simulink model "sync_baseline"  (R2025b)
settings: Solver=VariableStepAuto  StartTime=0.0  StopTime=10.0  RelTol=1e-3
values from neighbouring files (symbols this model uses):
  Dm = 1e-3    (= 0.001)    [foc_controlsystem_param.m]    (also in motor_param.m)
  Ki_id = wc_c*Rs    (= 380)    [foc_controlsystem_param.m]    (also in motor_param.m)
  Ki_iq = wc_c*Rs    (= 380)    [foc_controlsystem_param.m]    (also in motor_param.m)
  Ki_s = 0.041    [foc_controlsystem_param.m]    (also in motor_param.m)
  Kp_id = wc_c*Ld    (= 10)    [foc_controlsystem_param.m]    (also in motor_param.m)
  Kp_iq = wc_c*Lq    (= 20)    [foc_controlsystem_param.m]    (also in motor_param.m)
  Kp_s = 0.0014    [foc_controlsystem_param.m]    (also in motor_param.m)
  Ld = 0.01    [foc_controlsystem_param.m]    (also in motor_param.m)
  Lq = 0.02    [foc_controlsystem_param.m]    (also in motor_param.m)
  p = 2    [foc_controlsystem_param.m]    (also in motor_param.m)
  Phi = 0.1    [foc_controlsystem_param.m]    (also in motor_param.m)
libraries: fl_lib x60, nesl_utility x60, slpidlib x18, ee_lib x18, eeTransforms x12
(part 5 of 5)

== system sync_baseline/Subsystem5/Controller/FOC/VelocityController ==
  wmref : Inport
  wm : Inport  Port=2
  Gain : Gain  Gain=1/(3/2*p*Phi)
  PIDController : slpidlib/PID Controller  Controller=PI  Form=Parallel  TimeDomain=Continuous-time  UseExternalTs=off  SampleTime=-1  IntegratorMethod=Forward Euler  FilterMethod=Forward Euler  ControllerParametersSource=internal  P=Kp_s  I=Ki_s  UseKiTs=off  D=0  UseExternalDerivativeSource=off  N=100  UseFilter=on  TunerSelectOption=Transfer Function Based (PID Tuner App)  InitialConditionSource=internal  InitialConditionForIntegrator=0  InitialConditionForFilter=0  DifferentiatorICPrevScaledInput=0  ExternalReset=none  TrackingMode=off  Kt=1  LimitOutput=off  SatLimitsSource=internal  UpperSaturationLimit=inf  LowerSaturationLimit=-inf  LinearizeAsGain=on  AntiWindupMode=none  Kb=1  LimitIntegrator=off  UpperIntegratorSaturationLimit=inf  LowerIntegratorSaturationLimit=-inf  POutMin=[]  POutMax=[]  IOutMin=[]  IOutMax=[]  DOutMin=[]  DOutMax=[]  NOutMin=[]  NOutMax=[]  SumOutMin=[]  SumOutMax=[]  SaturationOutMin=[]  SaturationOutMax=[]  PParamMin=[]  PParamMax=[]  IParamMin=[]  IParamMax=[]  DParamMin=[]  DParamMax=[]  NParamMin=[]  NParamMax=[]  KbParamMin=[]  KbParamMax=[]  KtParamMin=[]  KtParamMax=[]  KbOutMin=[]  KbOutMax=[]  KtOutMin=[]  KtOutMax=[]  IntegratorOutMin=[]  IntegratorOutMax=[]  FilterOutMin=[]  FilterOutMax=[]  SumI1OutMin=[]  SumI1OutMax=[]  SumI2OutMin=[]  SumI2OutMax=[]  SumI3OutMin=[]  SumI3OutMax=[]  SumI4OutMin=[]  SumI4OutMax=[]  SumDOutMin=[]  SumDOutMax=[]  DifferentiatorOutMin=[]  DifferentiatorOutMax=[]  FilterDiffOutCoefMin=[]  FilterDiffOutCoefMax=[]  ReciprocalOutMin=[]  ReciprocalOutMax=[]  SumDenOutMin=[]  SumDenOutMax=[]  SumNumOutMin=[]  SumNumOutMax=[]  DivideOutMin=[]  DivideOutMax=[]  UdiffTsProdOutMin=[]  UdiffTsProdOutMax=[]  NTsProdOutMin=[]  NTsProdOutMax=[]  UintegralTsProdOutMin=[]  UintegralTsProdOutMax=[]  UngainTsProdOutMin=[]  UngainTsProdOutMax=[]  ClampingZeroOutDataTypeStr=Inherit: Inherit via back propagation  ClampingZeroOutMin=[]  ClampingZeroOutMax=[]  FilterDenConstantOutDataTypeStr=Inherit: Inherit via back propagation  FilterDenConstantOutMin=[]  FilterDenConstantOutMax=[]  PCopyOutDataTypeStr=Inherit: Inherit via back propagation  PCopyOutMin=[]  PCopyOutMax=[]  NCopyOutDataTypeStr=Inherit: Inherit via back propagation  NCopyOutMin=[]  NCopyOutMax=[]  IntegratorContinuousStateAttributes=''  IntegratorStateMustResolveToSignalObject=off  IntegratorRTWStateStorageClass=Auto  FilterContinuousStateAttributes=''  FilterStateMustResolveToSignalObject=off  FilterRTWStateStorageClass=Auto  ParallelPVariant=InternalParameters  IdealPVariant=Disabled  IVariant=InternalParameters  DVariant=Disabled  IntegratorVariant=Continuous  SatVariant=Disabled  AWVariant=Passthrough  PCopyVariant=Disabled  TRVariant=Disabled  FdbkBlocksVariant=Forward  IdealPFdbkVariant=Disabled  SatFdbkVariant=Disabled  DerivativeFilterVariant=Disabled  NVariant=Disabled  NCopyVariant=Disabled_SignalSpec  FilterICVariant=Disabled  IntegratorICVariant=InternalICs  ExternalResetVariant=Disabled  TRSumVariant=Passthrough  SumFdbkVariant=Disabled  SumVariant=Sum_PI  TsampFilterVariant=InternalTs  TsampNgainVariant=Passthrough  TsampIntegralVariant=Disabled_SignalSpec  ExternalSaturationOutDataTypeStr=Inherit: Same as second input  DerivativeSourceVariant=Disabled  PreIntVariant=InternalPreInt
  Sum : Sum  Inputs=|+-
  Iqref : Outport  VectorParamsAs1DForOutWhenUnconnected=off
  wires:
  PIDController/1 -> Gain/1
  Gain/1 -> Iqref/1
  wmref/1 -> Sum/1
  Sum/1 -> PIDController/1
  wm/1 -> Sum/2

== system sync_baseline/Subsystem5/Controller/FOC/abc2dq ==
  Iabc : Inport
  thetae : Inport  Port=2
  Demux1 : Demux  Outputs=3
  Park Transform : eeTransforms/Park Transform  AxisAlignment=D-axis  PowerInvariant=off
  Terminator : Terminator
  Id : Outport  VectorParamsAs1DForOutWhenUnconnected=off
  Iq : Outport  Port=2  VectorParamsAs1DForOutWhenUnconnected=off
  wires:
  Iabc/1 -> Park Transform/1
  thetae/1 -> Park Transform/2
  Demux1/3 -> Terminator/1
  Park Transform/1 -> Demux1/1
  Demux1/1 -> Id/1
  Demux1/2 -> Iq/1

== system sync_baseline/Subsystem5/Controller/FOC/dq2abc ==
  Vd : Inport
  Vq : Inport  Port=2
  thetae : Inport  Port=3
  Constant : Constant  Value=0
  Inverse Park Transform : eeTransforms/Inverse Park Transform  AxisAlignment=D-axis  PowerInvariant=off
  Mux : Mux  Inputs=3
  Vabc : Outport  VectorParamsAs1DForOutWhenUnconnected=off
  wires:
  thetae/1 -> Inverse Park Transform/2
  Constant/1 -> Mux/3
  Mux/1 -> Inverse Park Transform/1
  Vd/1 -> Mux/1
  Inverse Park Transform/1 -> Vabc/1
  Vq/1 -> Mux/2

== system sync_baseline/Subsystem5/Controller/FOC/thm2the ==
  thm : Inport
  Constant : Constant  Value=2*pi
  Mod : Math  Operator=mod  SignedPower=on
  PolePairs : Gain  Gain=p
  the : Outport  VectorParamsAs1DForOutWhenUnconnected=off
  wires:
  Constant/1 -> Mod/2
  PolePairs/1 -> Mod/1
  Mod/1 -> the/1
  thm/1 -> PolePairs/1

== system sync_baseline/Subsystem5/Controller/FOC/wm2we ==
  wm : Inport
  PolePairs : Gain  Gain=p
  we : Outport  VectorParamsAs1DForOutWhenUnconnected=off
  wires:
  wm/1 -> PolePairs/1
  PolePairs/1 -> we/1

== system sync_baseline/Subsystem/Controller/FOC/CurrentController/Decoupling ==
  note: VdFF = -Lq*Iq*we
  note: VqFF = Ld*Id*we + Phi*we
  Id : Inport
  Iq : Inport  Port=2
  we : Inport  Port=3
  Constant : Constant  Value=Lq
  Constant1 : Constant  Value=Ld
  Constant2 : Constant  Value=Phi
  Gain1 : Gain  Gain=-1
  Product{,1..3} (4 alike) : Product
  Sum : Sum  Inputs=|++
  VdFF : Outport  VectorParamsAs1DForOutWhenUnconnected=off
  VqFF : Outport  Port=2  VectorParamsAs1DForOutWhenUnconnected=off
  wires:
  we/1 -> Product3/2, Product2/2
  Product1/1 -> Sum/1
  Constant2/1 -> Sum/2
  Sum/1 -> Product2/1
  Constant1/1 -> Product1/2
  Id/1 -> Product1/1
  Iq/1 -> Product/1
  Constant/1 -> Product/2
  Product3/1 -> Gain1/1
  Product/1 -> Product3/1
  Gain1/1 -> VdFF/1
  Product2/1 -> VqFF/1

== system sync_baseline/Subsystem1/Controller/FOC/CurrentController/Decoupling ==
  note: VdFF = -Lq*Iq*we
  note: VqFF = Ld*Id*we + Phi*we
  Id : Inport
  Iq : Inport  Port=2
  we : Inport  Port=3
  Constant : Constant  Value=Lq
  Constant1 : Constant  Value=Ld
  Constant2 : Constant  Value=Phi
  Gain1 : Gain  Gain=-1
  Product{,1..3} (4 alike) : Product
  Sum : Sum  Inputs=|++
  VdFF : Outport  VectorParamsAs1DForOutWhenUnconnected=off
  VqFF : Outport  Port=2  VectorParamsAs1DForOutWhenUnconnected=off
  wires:
  we/1 -> Product3/2, Product2/2
  Product1/1 -> Sum/1
  Constant2/1 -> Sum/2
  Sum/1 -> Product2/1
  Constant1/1 -> Product1/2
  Id/1 -> Product1/1
  Iq/1 -> Product/1
  Constant/1 -> Product/2
  Product3/1 -> Gain1/1
  Product/1 -> Product3/1
  Gain1/1 -> VdFF/1
  Product2/1 -> VqFF/1

== system sync_baseline/Subsystem2/Controller/FOC/CurrentController/Decoupling ==
  note: VdFF = -Lq*Iq*we
  note: VqFF = Ld*Id*we + Phi*we
  Id : Inport
  Iq : Inport  Port=2
  we : Inport  Port=3
  Constant : Constant  Value=Lq
  Constant1 : Constant  Value=Ld
  Constant2 : Constant  Value=Phi
  Gain1 : Gain  Gain=-1
  Product{,1..3} (4 alike) : Product
  Sum : Sum  Inputs=|++
  VdFF : Outport  VectorParamsAs1DForOutWhenUnconnected=off
  VqFF : Outport  Port=2  VectorParamsAs1DForOutWhenUnconnected=off
  wires:
  we/1 -> Product3/2, Product2/2
  Product1/1 -> Sum/1
  Constant2/1 -> Sum/2
  Sum/1 -> Product2/1
  Constant1/1 -> Product1/2
  Id/1 -> Product1/1
  Iq/1 -> Product/1
  Constant/1 -> Product/2
  Product3/1 -> Gain1/1
  Product/1 -> Product3/1
  Gain1/1 -> VdFF/1
  Product2/1 -> VqFF/1

== system sync_baseline/Subsystem3/Controller/FOC/CurrentController/Decoupling ==
  note: VdFF = -Lq*Iq*we
  note: VqFF = Ld*Id*we + Phi*we
  Id : Inport
  Iq : Inport  Port=2
  we : Inport  Port=3
  Constant : Constant  Value=Lq
  Constant1 : Constant  Value=Ld
  Constant2 : Constant  Value=Phi
  Gain1 : Gain  Gain=-1
  Product{,1..3} (4 alike) : Product
  Sum : Sum  Inputs=|++
  VdFF : Outport  VectorParamsAs1DForOutWhenUnconnected=off
  VqFF : Outport  Port=2  VectorParamsAs1DForOutWhenUnconnected=off
  wires:
  we/1 -> Product3/2, Product2/2
  Product1/1 -> Sum/1
  Constant2/1 -> Sum/2
  Sum/1 -> Product2/1
  Constant1/1 -> Product1/2
  Id/1 -> Product1/1
  Iq/1 -> Product/1
  Constant/1 -> Product/2
  Product3/1 -> Gain1/1
  Product/1 -> Product3/1
  Gain1/1 -> VdFF/1
  Product2/1 -> VqFF/1

== system sync_baseline/Subsystem4/Controller/FOC/CurrentController/Decoupling ==
  note: VdFF = -Lq*Iq*we
  note: VqFF = Ld*Id*we + Phi*we
  Id : Inport
  Iq : Inport  Port=2
  we : Inport  Port=3
  Constant : Constant  Value=Lq
  Constant1 : Constant  Value=Ld
  Constant2 : Constant  Value=Phi
  Gain1 : Gain  Gain=-1
  Product{,1..3} (4 alike) : Product
  Sum : Sum  Inputs=|++
  VdFF : Outport  VectorParamsAs1DForOutWhenUnconnected=off
  VqFF : Outport  Port=2  VectorParamsAs1DForOutWhenUnconnected=off
  wires:
  we/1 -> Product3/2, Product2/2
  Product1/1 -> Sum/1
  Constant2/1 -> Sum/2
  Sum/1 -> Product2/1
  Constant1/1 -> Product1/2
  Id/1 -> Product1/1
  Iq/1 -> Product/1
  Constant/1 -> Product/2
  Product3/1 -> Gain1/1
  Product/1 -> Product3/1
  Gain1/1 -> VdFF/1
  Product2/1 -> VqFF/1

== system sync_baseline/Subsystem5/Controller/FOC/CurrentController/Decoupling ==
  note: VdFF = -Lq*Iq*we
  note: VqFF = Ld*Id*we + Phi*we
  Id : Inport
  Iq : Inport  Port=2
  we : Inport  Port=3
  Constant : Constant  Value=Lq
  Constant1 : Constant  Value=Ld
  Constant2 : Constant  Value=Phi
  Gain1 : Gain  Gain=-1
  Product{,1..3} (4 alike) : Product
  Sum : Sum  Inputs=|++
  VdFF : Outport  VectorParamsAs1DForOutWhenUnconnected=off
  VqFF : Outport  Port=2  VectorParamsAs1DForOutWhenUnconnected=off
  wires:
  we/1 -> Product3/2, Product2/2
  Product1/1 -> Sum/1
  Constant2/1 -> Sum/2
  Sum/1 -> Product2/1
  Constant1/1 -> Product1/2
  Id/1 -> Product1/1
  Iq/1 -> Product/1
  Constant/1 -> Product/2
  Product3/1 -> Gain1/1
  Product/1 -> Product3/1
  Gain1/1 -> VdFF/1
  Product2/1 -> VqFF/1

== matlab function sync_baseline/MATLAB Function ==
  data: w_vector input; w_ref_out output; w_ref_master input
function w_ref_out = Sync_Controller(w_vector, w_ref_master)
    %===== 参数设置 (来自 Stable1.m) =====
    % 邻接矩阵 L (假设5台电机)
    L = [0 0.6 0.7 0 0.8; 
         0.6 0 1.3 0.8 1.2; 
         0.7 1.3 0 1 0; 
         0 0.8 1 0 0.5; 
         0.8 1.2 0 0.5 0];
    
    % 控制增益 (对应代码中的 b)
    % 在实际工程中需根据电机惯量调试，建议从 0.01 开始尝试
    K_sync = 0.14; 
    
    %===== 核心算法实现 =====
    % 获取电机数量
    N = length(w_vector);
    
    % 初始化输出
    delta_w = zeros(N, 1);
    
    % 计算耦合项 (对应代码中的 b*sum(L(i,j)*(x_j - x_i)))
    % 注意：Matlab索引从1开始
    for i = 1:N
        sum_coupling = 0;
        for j = 1:N
            % 耦合项：邻居状态差 * 邻接权重
            sum_coupling = sum_coupling + L(i,j) * (w_vector(j) - w_vector(i));
        end
        % 累加得到每台电机的修正量
        delta_w(i) = K_sync * sum_coupling;
    end
    
    %===== 输出计算 =====
    % 最终参考 = 主参考 + 同步修正量
    w_ref_out = w_ref_master + delta_w';
end

== matlab function sync_baseline/MATLAB Function1 ==
  data: w input; error output; w_ref input
function error = err_cul(w,w_ref)
err = zeros(length(w));
for i = 1:length(w)
    err(i) = w_ref - w(i);
end
error = norm(err);
